simulink model "control_03_attitude"  (R2020a)
settings: Solver=FixedStepAuto  StartTime=0.0  StopTime=10.0  RelTol=1e-3
settings Model: Creator=Bayram  LastModifiedBy=Bayram

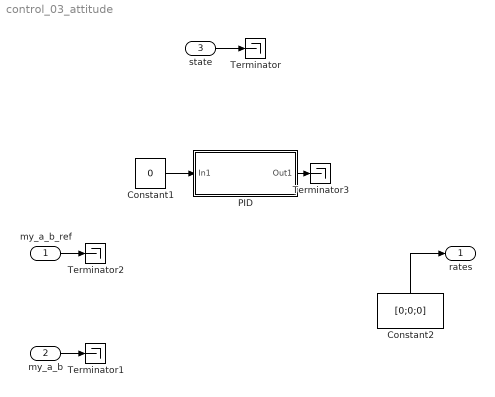
== system control_03_attitude ==
  my_a_b_ref : Inport  OutDataTypeStr=single  PortDimensions=3
  my_a_b : Inport  Port=2  OutDataTypeStr=single  PortDimensions=3
  state : Inport  Port=3  OutDataTypeStr=Bus:fmBus
  Constant1 : Constant  Value=0  OutDataTypeStr=single
  Constant2 : Constant  Value=[0;0;0]  OutDataTypeStr=single
  PID : Subsystem
  Terminator{,1..3} (4 alike) : Terminator
  rates : Outport  PortDimensions=3
  wires:
  state/1 -> Terminator/1
  Constant2/1 -> rates/1
  my_a_b/1 -> Terminator1/1
  my_a_b_ref/1 -> Terminator2/1
  Constant1/1 -> PID/1(In1)
  PID/1(Out1) -> Terminator3/1

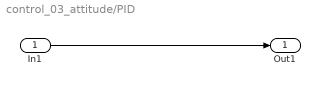
== system control_03_attitude/PID ==
  In1 : Inport
  Out1 : Outport
  wires:
  In1/1 -> Out1/1
